simulink model "Controller"  (R2021b)
settings: Solver=FixedStepAuto  StartTime=0.0  StopTime=60  RelTol=1e-3  EnableMultiTasking=on
libraries: simulink x6, legoev3lib x6, dspsigops x3, simulink_extras x2
settings Model: ExtModeTrigDuration=2  Creator=s142  LastModifiedBy=s142
settings SolverCC: PositivePriorityOrder=on
settings OptimizationCC: EnhancedBackFolding=on  PassReuseOutputArgsAs=Individual arguments  ZeroExternalMemoryAtStartup=off  ZeroInternalMemoryAtStartup=off  MaxStackSize=64  OptimizeBlockOrder=speed  DifferentSizesBufferReuse=on  OptimizationCustomize=off  EfficientTunableParamExpr=on
settings DebuggingCC: ParameterTunabilityLossMsg=error
settings HardwareCC: ProdBitPerPointer=32  ProdBitPerSizeT=32  ProdBitPerPtrDiffT=32  ProdLargestAtomicInteger=Long  ProdWordSize=32  ProdHWDeviceType=ARM Compatible->ARM 9
settings SFSimCC: MATLABDynamicMemAlloc=off
settings RTWCC: Description=Embedded Coder  SystemTargetFile=ert.tlc  HardwareBoard=LEGO MINDSTORMS EV3  TLCOptions="-aInlineSetEventsForThisBaseRateFcn=TLC_FALSE -aSuppressMultiTaskScheduler=TLC_FALSE  -aRateBasedStepFcn=0"  TemplateMakefile=ert_default_tmf  Toolchain=Sourcery G++ Lite v2009q3
settings CodeAppCC: ForceParamTrailComments=on  IgnoreCustomStorageClasses=off  OperatorAnnotations=on  SimulinkDataObjDesc=on  SFDataObjDesc=on  InsertBlockDesc=on
settings ERTTargetCC: SupportContinuousTime=on  SupportVariableSizeSignals=on  ExtModeTransport=2  ExtModeStaticAlloc=on  ExtModeMexFile=ext_xcp  ExtModeIntrfLevel=Level2 - Open

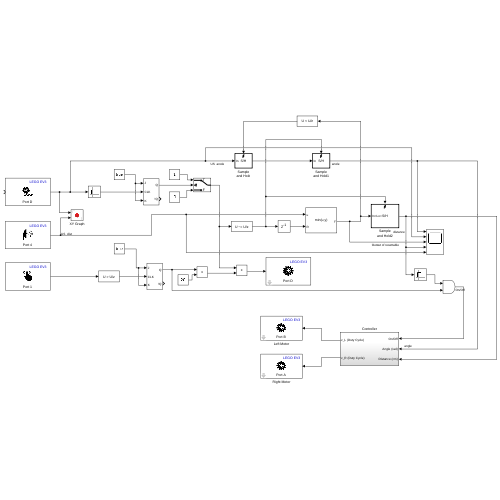
[thumbnail: Simulink's stored preview of the top-level diagram]
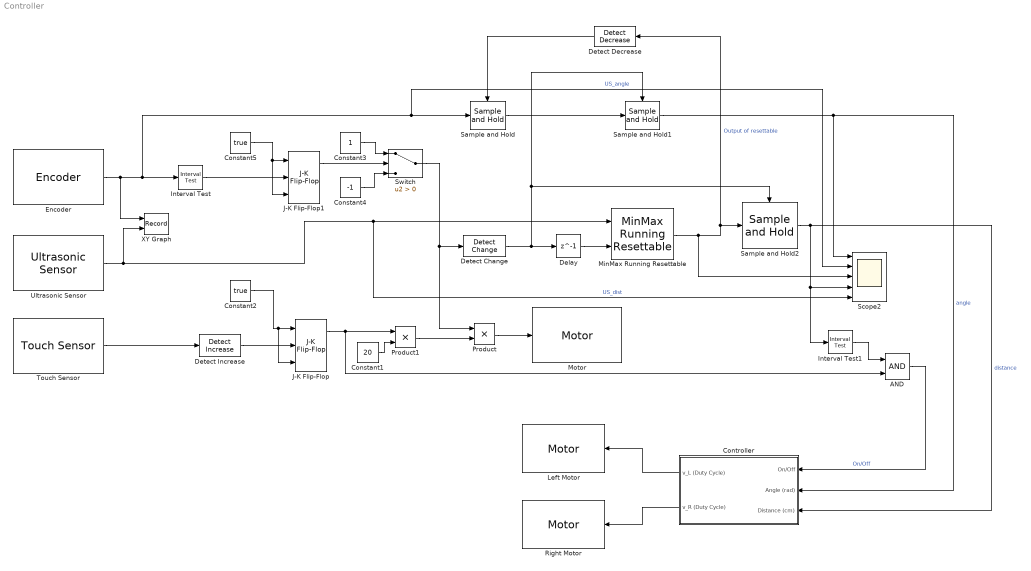
== system Controller ==
  AND : Logic  IconShape=distinctive  AllPortsSameDT=off  OutDataTypeStr=boolean
  Constant1 : Constant  Value=20
  Constant2 : Constant  Value=true  OutDataTypeStr=boolean
  Constant3 : Constant
  Constant4 : Constant  Value=-1
  Constant5 : Constant  Value=true  OutDataTypeStr=boolean
  Controller : Subsystem
  Delay : Delay  DelayLength=1
  Detect Change : simulink/Logic and Bit Operations/Detect Change  vinit=1  OutDataTypeStr=boolean
  Detect Decrease : simulink/Logic and Bit Operations/Detect Decrease  vinit=200  OutDataTypeStr=boolean
  Detect Increase : simulink/Logic and Bit Operations/Detect Increase  vinit=0.0  OutDataTypeStr=boolean
  Encoder : legoev3lib/Encoder  portNumber=D  opMode=Reset by external signal  sampleTime=0.01
      settings: SourceProductBaseCode=LEGOEV3
  Interval Test : simulink/Logic and Bit Operations/Interval Test  IntervalClosedRight=on  uplimit=60  IntervalClosedLeft=on  lowlimit=-60  OutDataTypeStr=boolean
  Interval Test1 : simulink/Logic and Bit Operations/Interval Test  IntervalClosedRight=on  uplimit=150  IntervalClosedLeft=on  lowlimit=25  OutDataTypeStr=boolean
  J-K Flip-Flop : simulink_extras/Flip Flops/J-K Flip-Flop  initial_condition=0
  J-K Flip-Flop1 : simulink_extras/Flip Flops/J-K Flip-Flop  initial_condition=0
  Left Motor : legoev3lib/Motor  sportNumber=B  sstopAction=Brake
  MinMax Running Resettable : simulink/Math Operations/MinMax Running Resettable  Function=min  vinit=200
  Motor : legoev3lib/Motor  sportNumber=D  sstopAction=Brake
  Product : Product
  Product1 : Product
  Right Motor : legoev3lib/Motor  sportNumber=A  sstopAction=Brake
  Sample and Hold : dspsigops/Sample and Hold  trig=Rising edge  initCond=0  latchinput=off
  Sample and Hold1 : dspsigops/Sample and Hold  trig=Rising edge  initCond=0  latchinput=off
  Sample and Hold2 : dspsigops/Sample and Hold  trig=Rising edge  initCond=0  latchinput=on
  Scope2 : Scope  NumInputPorts=5
  Switch : Switch  Criteria=u2 > Threshold
  Touch Sensor : legoev3lib/Touch Sensor  portNumber=1  sampleTime=0.01
      settings: SourceProductBaseCode=LEGOEV3
  Ultrasonic Sensor : legoev3lib/Ultrasonic Sensor  PortNumber=4  sampleTime=0.01
      settings: SourceProductBaseCode=LEGOEV3
  XY Graph : Record  FileSettingsInternal="{\"entries\":[{\"content\":{\"excelSettings\":{\"content\":{},\"type\":\"Streamout.ExcelSettings\"}},\"type\":\"Streamout.FileSettingStorage\",\"uuid\":\"50f50f7a-dfcd-414a-8b4a-e8b5aee4ef2a\"}],\"packageUris\":[\"http://schema.mathworks.com/mf0/streamout_blocks/R2020a\"],\"version\":\"1.0\"}"  Layout=[1 1]  SignalsInternal="{\"entries\":[{\"content\":{\"signals\":[{\"content\":{\"blockPath\":[\"exercise_34/XY Graph\"],\"channel\":[],\"dimensions\":[1],\"domain\":\"exercise_34/XY Graph\",\"lineColor\":\"#ff6929\",\"plots\":[],\"port\":2,\"sid\":[\"18\"],\"signalID\":143223,\"signalName\":\"US_dist\"},\"type\":\"RecordBlkView.Signal\",\"uuid\":\"9f4c7783-9e64-4194-b0c8-e27f466223ce\"},{\"content\":{\"blockPath\":[\"exercise_34/XY Graph\"],\"channel\":[],\"dimensions\":[1],\"domain\":\"exercise_34/XY Graph\",\"lineColor\":\"#d95319\",\"plots\":[],\"port\":1,\"sid\":[\"18\"],\"signalID\":143251,\"signalName\":\"US_angle\"},\"type\":\"RecordBlkView.Signal\",\"uuid\":\"8fa6fd90-3c0c-47df-8306-6f92436ad4df\"}]},\"type\":\"RecordBlkView.InputSignals\",\"uuid\":\"913f0c80-a840-4b5b-8a5a-faa2ee1028a1\"}],\"packageUris\":[\"http://schema.mathworks.com/mf0/streamout_blocks/R2020a\"],\"version\":\"1.0\"}"  VisualizationBindings="{\"xyplotplugin\":{\"info\":[{\"series\":[],\"subplotID\":1}]}}"  CompatibilityTag=XY
  wires:
  J-K Flip-Flop/1 -> AND/2, Product1/1
  Encoder/1 -> Scope2/2, Sample and Hold/1, Interval Test/1, XY Graph/1  "US_angle"
  Constant2/1 -> J-K Flip-Flop/3, J-K Flip-Flop/1
  Constant1/1 -> Product1/2
  Product1/1 -> Product/2
  Ultrasonic Sensor/1 -> Scope2/5, MinMax Running Resettable/1, XY Graph/2  "US_dist"
  Constant5/1 -> J-K Flip-Flop1/3, J-K Flip-Flop1/1
  Touch Sensor/1 -> Detect Increase/1
  Constant4/1 -> Switch/3
  J-K Flip-Flop1/1 -> Switch/2
  Product/1 -> Motor/1
  Constant3/1 -> Switch/1
  Switch/1 -> Detect Change/1, Product/1
  Detect Increase/1 -> J-K Flip-Flop/2
  Interval Test/1 -> J-K Flip-Flop1/2
  Detect Change/1 -> Sample and Hold2/Trigger, Sample and Hold1/Trigger, Delay/1
  MinMax Running Resettable/1 -> Detect Decrease/1, Sample and Hold2/1, Scope2/3  "Output of resettable"
  Sample and Hold2/1 -> Interval Test1/1, Scope2/4, Controller/3(Distance (cm))  "distance"
  Interval Test1/1 -> AND/1
  Sample and Hold/1 -> Sample and Hold1/1
  AND/1 -> Controller/1(On/Off)  "On/Off"
  Sample and Hold1/1 -> Scope2/1, Controller/2(Angle (rad))  "angle"
  Detect Decrease/1 -> Sample and Hold/Trigger
  Delay/1 -> MinMax Running Resettable/2
  Controller/1(v_L (Duty Cycle)) -> Left Motor/1
  Controller/2(v_R (Duty Cycle)) -> Right Motor/1

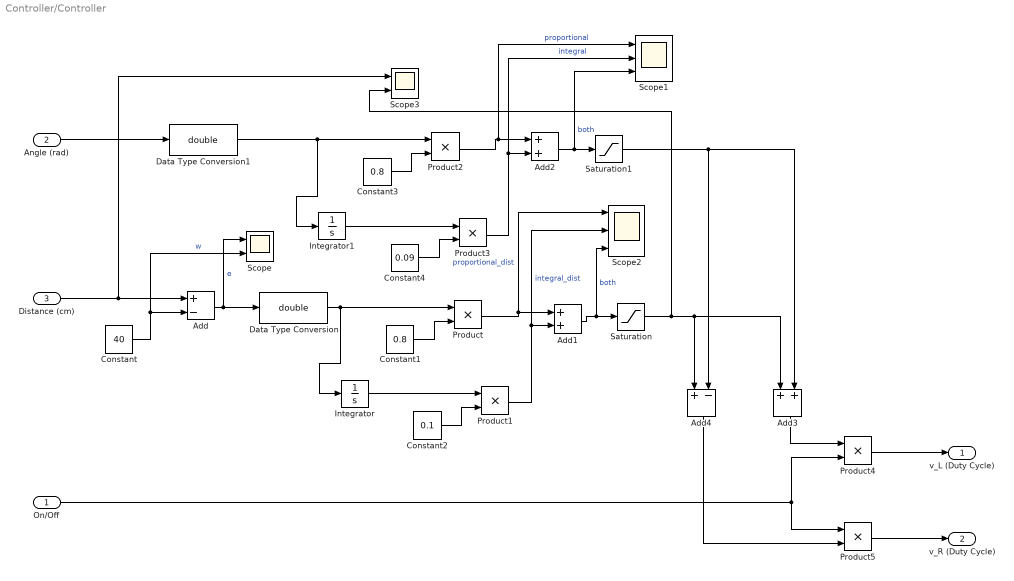
== system Controller/Controller ==
  On/Off : Inport
  Angle (rad) : Inport  Port=2
  Distance (cm) : Inport  Port=3
  Add : Sum  Inputs=+-
  Add1 : Sum
  Add2 : Sum
  Add3 : Sum
  Add4 : Sum  Inputs=+-
  Constant : Constant  Value=40
  Constant1 : Constant  Value=0.8
  Constant2 : Constant  Value=0.1
  Constant3 : Constant  Value=0.8
  Constant4 : Constant  Value=0.09
  Data Type Conversion : DataTypeConversion  OutDataTypeStr=double
  Data Type Conversion1 : DataTypeConversion  OutDataTypeStr=double
  Integrator : Integrator
  Integrator1 : Integrator
  Product{,1..5} (6 alike) : Product
  Saturation : Saturate  UpperLimit=100  LowerLimit=-100
  Saturation1 : Saturate  UpperLimit=50  LowerLimit=-50
  Scope : Scope  NumInputPorts=2
  Scope1 : Scope  NumInputPorts=3
  Scope2 : Scope  NumInputPorts=3
  Scope3 : Scope  NumInputPorts=2
  v_L (Duty Cycle) : Outport
  v_R (Duty Cycle) : Outport  Port=2
  wires:
  Add4/1 -> Product5/2
  Product2/1 -> Scope1/1, Add2/1  "proportional"
  Saturation1/1 -> Add4/2, Add3/2
  Data Type Conversion1/1 -> Integrator1/1, Product2/1
  On/Off/1 -> Product5/1, Product4/2
  Angle (rad)/1 -> Data Type Conversion1/1
  Add2/1 -> Scope1/3, Saturation1/1  "both"
  Constant/1 -> Add/2, Scope/2  "w"
  Product1/1 -> Scope2/2, Add1/2  "integral_dist"
  Constant1/1 -> Product/2
  Data Type Conversion/1 -> Integrator/1, Product/1
  Constant3/1 -> Product2/2
  Add1/1 -> Scope2/3, Saturation/1  "both"
  Constant2/1 -> Product1/2
  Distance (cm)/1 -> Scope3/1, Add/1
  Add/1 -> Scope/1, Data Type Conversion/1  "e"
  Integrator1/1 -> Product3/1
  Add3/1 -> Product4/1
  Product3/1 -> Scope1/2, Add2/2  "integral"
  Integrator/1 -> Product1/1
  Constant4/1 -> Product3/2
  Product4/1 -> v_L (Duty Cycle)/1
  Saturation/1 -> Scope3/2, Add3/1, Add4/1
  Product5/1 -> v_R (Duty Cycle)/1
  Product/1 -> Scope2/1, Add1/1  "proportional_dist"
